simulink model "calibration_valves"  (R2026a)
settings: Solver=VariableStepAuto  StopTime=inf
InitFcn:
  | coefficients = [0,coefficients];
StopFcn:
  | az = out.az;
  | save(fullfile('calibration_data','az_calibration.mat'),'az');
settings Model: Creator=user  LastModifiedBy=jinyu

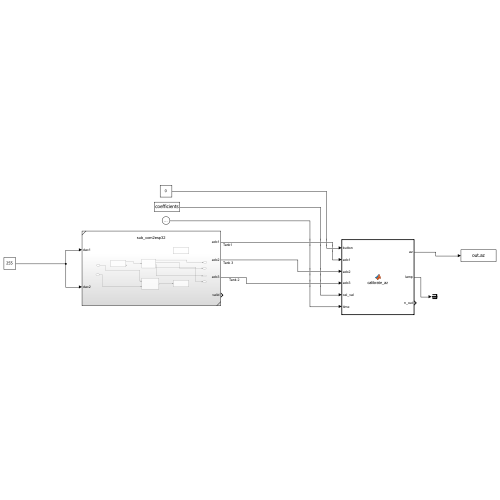
[thumbnail: Simulink's stored preview of the top-level diagram]
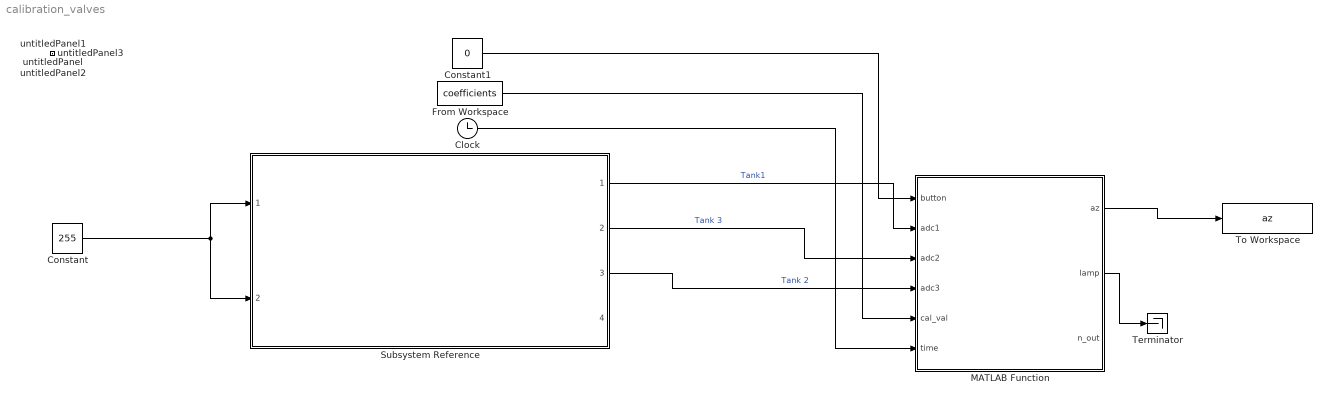
== system calibration_valves ==
  Clock : Clock
  Constant : Constant  Value=255
  Constant1 : Constant  Value=0
  From Workspace : FromWorkspace  VariableName=coefficients  SampleTime=-1
  MATLAB Function : MATLAB Function  TreatAsAtomicUnit=on
  Subsystem Reference : Subsystem  ReferencedSubsystem=sub_com2esp32
  Terminator : Terminator
  To Workspace : ToWorkspace  VariableName=az  SampleTime=-1
      settings: MaxDataPoints=1
  untitledPanel : Subsystem  Tag=HiddenForWebPanel  IsWebBlockPanel=on
  untitledPanel1 : Subsystem  Tag=HiddenForWebPanel  IsWebBlockPanel=on
  untitledPanel2 : Subsystem  Tag=HiddenForWebPanel  IsWebBlockPanel=on
  untitledPanel3 : Subsystem  Tag=HiddenForWebPanel  IsWebBlockPanel=on
  wires:
  Subsystem Reference/1 -> MATLAB Function/2(adc1)  "Tank1"
  MATLAB Function/1(az) -> To Workspace/1
  Constant/1 -> Subsystem Reference/2, Subsystem Reference/1
  From Workspace/1 -> MATLAB Function/5(cal_val)
  Clock/1 -> MATLAB Function/6(time)
  Constant1/1 -> MATLAB Function/1(button)
  Subsystem Reference/2 -> MATLAB Function/3(adc2)  "Tank 3"
  Subsystem Reference/3 -> MATLAB Function/4(adc3)  "Tank 2"
  MATLAB Function/2(lamp) -> Terminator/1

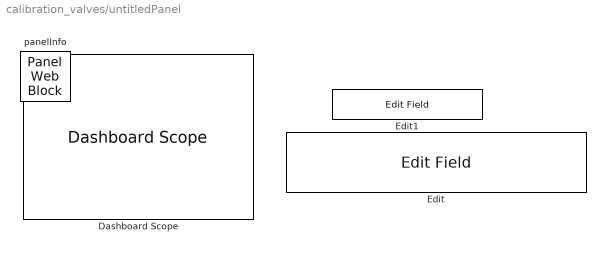
== system calibration_valves/untitledPanel ==
  Dashboard Scope : DashboardScope  Tag=HiddenForWebPanel  PanelInfo="{\"height\":195,\"left\":22,\"panelId\":\"panelId-0a8f6d05-5e0e-4052-8464-4cdde78ccbfe\",\"top\":22,\"type\":\"panelChild\",\"version\":\"2019b\",\"width\":271,\"zIndex\":1500002}"  FontColor=[0.0, 0.0, 0.0]
  Edit : EditField  Tag=HiddenForWebPanel  PanelInfo="{\"height\":25,\"left\":322,\"panelId\":\"panelId-0a8f6d05-5e0e-4052-8464-4cdde78ccbfe\",\"top\":100,\"type\":\"panelChild\",\"version\":\"2019b\",\"width\":181,\"zIndex\":1500006}"  LabelPosition=Hide  ShowInitialText=on  Alignment=Center
  Edit1 : EditField  Tag=HiddenForWebPanel  PanelInfo="{\"height\":30,\"left\":327,\"panelId\":\"panelId-0a8f6d05-5e0e-4052-8464-4cdde78ccbfe\",\"top\":53,\"type\":\"panelChild\",\"version\":\"2019b\",\"width\":150,\"zIndex\":1500004}"  LabelPosition=Hide  ShowInitialText=on  Alignment=Center
  panelInfo : PanelWebBlock  Tag=HiddenForWebPanel  PanelInfo="{\"compacted\":false,\"height\":362,\"isActiveTab\":false,\"left\":183,\"name\":\"Panel\",\"panelId\":\"panelId-0a8f6d05-5e0e-4052-8464-4cdde78ccbfe\",\"popoutData\":{\"height\":495,\"left\":546,\"maximized\":false,\"top\":827,\"width\":618},\"popoutMode\":\"windowHidden\",\"tabIndex\":0,\"tabbedSetId\":\"tabbedSet4972758365\",\"top\":737,\"type\":\"panel\",\"version\":\"2019b\",\"visible\":false,\"width\":602,\"zIndex\":1500002}"  PanelSnapshot=<binary blob, 20028 chars, not shown>

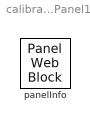
== system calibration_valves/untitledPanel1 ==
  panelInfo : PanelWebBlock  Tag=HiddenForWebPanel  PanelInfo="{\"compacted\":false,\"height\":362,\"isActiveTab\":true,\"left\":183,\"name\":\"Panel1\",\"panelId\":\"panelId-b2ee2f41-7720-49f1-b51a-3062c351f597\",\"popoutData\":{\"height\":495,\"left\":546,\"maximized\":false,\"top\":827,\"width\":618},\"popoutMode\":\"windowHidden\",\"tabIndex\":1,\"tabbedSetId\":\"tabbedSet4972758365\",\"top\":737,\"type\":\"panel\",\"version\":\"2019b\",\"visible\":true,\"width\":602,\"zIndex\":1500004}"

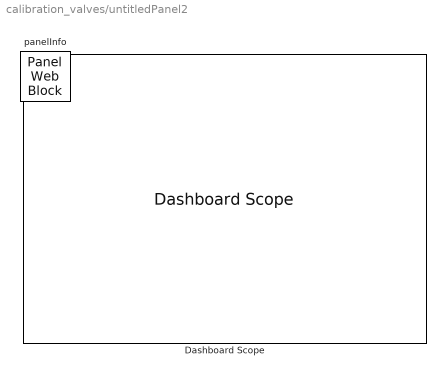
== system calibration_valves/untitledPanel2 ==
  Dashboard Scope : DashboardScope  Tag=HiddenForWebPanel  PanelInfo="{\"height\":289,\"left\":18,\"panelId\":\"panelId-8ba459e9-7eb9-43d1-9a8b-2b7bff5a2d5c\",\"top\":18,\"type\":\"panelChild\",\"version\":\"2019b\",\"width\":403,\"zIndex\":1500002}"  FontColor=[0.0, 0.0, 0.0]
  panelInfo : PanelWebBlock  Tag=HiddenForWebPanel  PanelInfo="{\"compacted\":false,\"height\":329,\"isActiveTab\":true,\"left\":1320,\"name\":\"Panel2\",\"panelId\":\"panelId-8ba459e9-7eb9-43d1-9a8b-2b7bff5a2d5c\",\"popoutData\":{\"height\":440,\"left\":1683,\"maximized\":false,\"top\":822,\"width\":459},\"popoutMode\":\"windowHidden\",\"tabIndex\":0,\"tabbedSetId\":\"tabbedSet1724704130\",\"top\":710,\"type\":\"panel\",\"version\":\"2019b\",\"visible\":true,\"width\":443,\"zIndex\":1500006}"  PanelSnapshot=<binary blob, 75208 chars, not shown>

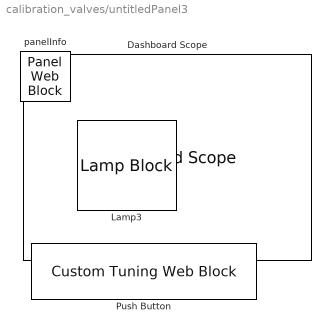
== system calibration_valves/untitledPanel3 ==
  Dashboard Scope : DashboardScope  Tag=HiddenForWebPanel  PanelInfo="{\"height\":461,\"left\":236,\"panelId\":\"panelId-037cc253-1a0e-430c-bfc3-d197bdfa8fb6\",\"top\":13,\"type\":\"panelChild\",\"version\":\"2019b\",\"width\":556,\"zIndex\":1500002}"  FontColor=[0.0, 0.0, 0.0]
  Lamp3 : LampBlock  Tag=HiddenForWebPanel  PanelInfo="{\"height\":68,\"left\":30,\"panelId\":\"panelId-037cc253-1a0e-430c-bfc3-d197bdfa8fb6\",\"top\":30,\"type\":\"panelChild\",\"version\":\"2019b\",\"width\":79,\"zIndex\":1500014}"  LabelPosition=Hide  DefaultColor=[192.0, 192.0, 192.0]
  Push Button : CustomTuningWebBlock  Tag=HiddenForWebPanel  PanelInfo="{\"height\":52,\"left\":27,\"panelId\":\"panelId-037cc253-1a0e-430c-bfc3-d197bdfa8fb6\",\"top\":105,\"type\":\"panelChild\",\"version\":\"2019b\",\"width\":209,\"zIndex\":1500008}"  LabelPosition=Hide  ShowInitialText=on  Configuration="{\"components\":[{\"name\":\"BackgroundImageComponent\",\"settings\":{\"image\":{\"size\":[0,0],\"src\":\"default\",\"srcOrientation\":\"horizontal\"},\"position\":[0,0,1,1],\"scaleMode\":\"0\"}},{\"name\":\"ButtonStateComponent\",\"settings\":{\"buttonType\":\"momentary\",\"clickFcn\":\"\",\"image\":{\"size\":[180,45],\"srcOrientation\":\"Right\"},\"latched\":false,\"offValue\":[],\"onValue\":1,\"position\":[0,0,1,1],\"pressDelay\":500,\"pressFcn\":\"\",\"repeatInterval\":0,\"states\":[{\"horizontalAlignment\":\"center\",\"image\":{\"position\":[0.05,0.015,0.98,0.9],\"size\":[0.98,0.9],\"src\":\"data:image\\/svg+xml;base64,PHN2ZyB4bWxucz0iaHR0cDovL3d3dy53My5vcmcvMjAwMC9zdmciIHhtbG5zOnhsaW5rPSJodHRwOi8vd3d3LnczLm9yZy8xOTk5L3hsaW5rIiB2aWV3Qm94PSIwIDAgMTc3LjI1IDQwLjg4Ij48ZGVmcz48c3R5bGU+LmNscy0xe2ZpbGw6dXJsKCNyYWRpYWwtZ3JhZGllbnQpO30uY2xzLTJ7ZmlsbDp1cmwoI2xpbmVhci1ncmFkaWVudCk7fS5jbHMtM3tmaWxsOnVybCgjbGluZWFyLWdyYWRpZW50LTIpO308L3N0eWxlPjxyYWRpYWxHcmFkaWVudCBpZD0icmFkaWFsLWdyYWRpZW50IiBjeD0iOTAuMDkiIGN5PSIyMi42NiIgcj0i ...(+2212 chars)\",\"srcOrientation\":\"Right\"},\"label\":{\"color\":[1,1,0.78,1],\"icon\":{\"size\":[1.2,1.2],\"src\":\"data:image\\/svg+xml;base64,PHN2ZyBpZD0iT2ZmIiB4bWxucz0iaHR0cDovL3d3dy53My5vcmcvMjAwMC9zdmciIHhtbG5zOnhsaW5rPSJodHRwOi8vd3d3LnczLm9yZy8xOTk5L3hsaW5rIiB2aWV3Qm94PSIwIDAgNTAgNTAiPjxkZWZzPjxzdHlsZT4uY2xzLTF7ZmlsbDojN2Y4MDgwO3N0cm9rZTojMjcyNjI2O3N0cm9rZS1taXRlcmxpbWl0OjEwO3N0cm9rZS13aWR0aDozcHg7fS5jbHMtMntmaWxsOnVybCgjbGluZWFyLWdyYWRpZW50KTt9PC9zdHlsZT48bGluZWFyR3JhZGllbnQgaWQ9ImxpbmVhci1ncmFkaWVudCIgeDE9IjI1IiB5MT0iOSIgeDI9IjI1IiB5Mj0iMzciIGdyYWRpZW50VW5pdHM9InVzZXJTcGFjZU9uVXNlIj48c3RvcCBvZmZzZXQ9IjAiIHN0b3AtY29sb3I9IiNmZmYiIHN0b3Atb3BhY2l0eT0iMC43NSIvPjxzdG9wIG9mZnNldD0iMSIgc3RvcC1jb2xvcj0iI2ZmZiIgc3RvcC1vcGFjaXR5PSIwIi8+PC9saW5lYXJHcmFkaWVudD48L2RlZnM+PGNpcmNsZSBjbGFzcz0iY2xzLTEiIGN4PSIyNSIgY3k9IjI1IiByPSIyMCIvPjxjaXJjbGUgY2xhc3M9ImNscy0yIiBjeD0iMjUiIGN5PSIyMyIgcj0iMTQiLz48L3N2Zz4=\",\"srcOrientation\":\"Right\"},\"iconOffset\":0,\"iconPlacement\":\"left\",\"opacity\":1,\"show\":true,\"text\":{\"content\":\"Button\",\"font\":\"Helvetica\"}},\"labelOffset\":[-0.025,0],\"verticalAlignment\":\"middle\"},{\"horizontalAlignment\":\"center\",\"image\":{\"position\":[0.05,0.015,0.98,0.9],\"size\":[0.98,0.9],\"src\":\"data:image\\/svg+xml;base64,PHN2ZyB4bWxucz0iaHR0cDovL3d3dy53My5vcmcvMjAwMC9zdmciIHhtbG5zOnhsaW5rPSJodHRwOi8vd3d3LnczLm9yZy8xOTk5L3hsaW5rIiB2aWV3Qm94PSIwIDAgMTc3LjI1IDQwLjg4Ij48ZGVmcz48c3R5bGU+LmNscy0xe2ZpbGw6dXJsKCNyYWRpYWwtZ3JhZGllbnQpO30uY2xzLTJ7ZmlsbDp1cmwoI2xpbmVhci1ncmFkaWVudCk7fS5jbHMtM3tmaWxsOnVybCgjbGluZWFyLWdyYWRpZW50LTIpO308L3N0eWxlPjxyYWRpYWxHcmFkaWVudCBpZD0icmFkaWFsLWdyYWRpZW50IiBjeD0iOTAuMDkiIGN5PSIyMi42NiIgcj0i ...(+2216 chars)\",\"srcOrientation\":\"Right\"},\"label\":{\"color\":[1,1,0.78,1],\"icon\":{\"size\":[1.2,1.2],\"src\":\"data:image\\/svg+xml;base64,PHN2ZyB4bWxucz0iaHR0cDovL3d3dy53My5vcmcvMjAwMC9zdmciIHhtbG5zOnhsaW5rPSJodHRwOi8vd3d3LnczLm9yZy8xOTk5L3hsaW5rIiB2aWV3Qm94PSIwIDAgNTAgNTAiPjxkZWZzPjxzdHlsZT4uY2xzLTF7ZmlsbDojNmFiZDQ1O3N0cm9rZTojMjcyNjI2O3N0cm9rZS1taXRlcmxpbWl0OjEwO3N0cm9rZS13aWR0aDozcHg7fS5jbHMtMntmaWxsOnVybCgjbGluZWFyLWdyYWRpZW50KTt9PC9zdHlsZT48bGluZWFyR3JhZGllbnQgaWQ9ImxpbmVhci1ncmFkaWVudCIgeDE9IjI1IiB5MT0iOSIgeDI9IjI1IiB5Mj0iMzciIGdyYWRpZW50VW5pdHM9InVzZXJTcGFjZU9uVXNlIj48c3RvcCBvZmZzZXQ9IjAiIHN0b3AtY29sb3I9IiNmZmYiIHN0b3Atb3BhY2l0eT0iMC43NSIvPjxzdG9wIG9mZnNldD0iMSIgc3RvcC1jb2xvcj0iI2ZmZiIgc3RvcC1vcGFjaXR5PSIwIi8+PC9saW5lYXJHcmFkaWVudD48L2RlZnM+PGcgaWQ9Ik9uIj48Y2lyY2xlIGNsYXNzPSJjbHMtMSIgY3g9IjI1IiBjeT0iMjUiIHI9IjIwIi8+PGNpcmNsZSBjbGFzcz0iY2xzLTIiIGN4PSIyNSIgY3k9IjIzIiByPSIxNCIvPjwvZz48L3N2Zz4=\",\"srcOrientation\":\"Right\"},\"iconOffset\":0,\"iconPlacement\":\"left\",\"opacity\":1,\"show\":true,\"text\":{\"content\":\"Button\",\"font\":\"Helvetica\"}},\"labelOffset\":[0,0],\"verticalAlignment\":\"middle\"},{\"horizontalAlignment\":\"center\",\"image\":{\"position\":[0.05,0.015,0.98,0.9],\"size\":[0.98,0.9],\"src\":\"data:image\\/svg+xml;base64,PHN2ZyB4bWxucz0iaHR0cDovL3d3dy53My5vcmcvMjAwMC9zdmciIHhtbG5zOnhsaW5rPSJodHRwOi8vd3d3LnczLm9yZy8xOTk5L3hsaW5rIiB2aWV3Qm94PSIwIDAgMTc3LjI1IDQwLjg4Ij48ZGVmcz48c3R5bGU+LmNscy0xe2ZpbGw6dXJsKCNyYWRpYWwtZ3JhZGllbnQpO30uY2xzLTJ7ZmlsbDp1cmwoI2xpbmVhci1ncmFkaWVudCk7fS5jbHMtM3tmaWxsOnVybCgjbGluZWFyLWdyYWRpZW50LTIpO308L3N0eWxlPjxyYWRpYWxHcmFkaWVudCBpZD0icmFkaWFsLWdyYWRpZW50IiBjeD0iOTAuMDkiIGN5PSIyMi42NiIgcj0i ...(+2212 chars)\",\"srcOrientation\":\"Right\"},\"label\":{\"color\":[1,1,0.78,1],\"icon\":{\"size\":[1.2,1.2],\"src\":\"data:image\\/svg+xml;base64,PHN2ZyB4bWxucz0iaHR0cDovL3d3dy53My5vcmcvMjAwMC9zdmciIHhtbG5zOnhsaW5rPSJodHRwOi8vd3d3LnczLm9yZy8xOTk5L3hsaW5rIiB2aWV3Qm94PSIwIDAgNTAgNTAiPjxkZWZzPjxzdHlsZT4uY2xzLTF7ZmlsbDojNmFiZDQ1O3N0cm9rZTojMjcyNjI2O3N0cm9rZS1taXRlcmxpbWl0OjEwO3N0cm9rZS13aWR0aDozcHg7fS5jbHMtMntmaWxsOnVybCgjbGluZWFyLWdyYWRpZW50KTt9PC9zdHlsZT48bGluZWFyR3JhZGllbnQgaWQ9ImxpbmVhci1ncmFkaWVudCIgeDE9IjI1IiB5MT0iOSIgeDI9IjI1IiB5Mj0iMzciIGdyYWRpZW50VW5pdHM9InVzZXJTcGFjZU9uVXNlIj48c3RvcCBvZmZzZXQ9IjAiIHN0b3AtY29sb3I9IiNmZmYiIHN0b3Atb3BhY2l0eT0iMC43NSIvPjxzdG9wIG9mZnNldD0iMSIgc3RvcC1jb2xvcj0iI2ZmZiIgc3RvcC1vcGFjaXR5PSIwIi8+PC9saW5lYXJHcmFkaWVudD48L2RlZnM+PGcgaWQ9Ik9uIj48Y2lyY2xlIGNsYXNzPSJjbHMtMSIgY3g9IjI1IiBjeT0iMjUiIHI9IjIwIi8+PGNpcmNsZSBjbGFzcz0iY2xzLTIiIGN4PSIyNSIgY3k9IjIzIiByPSIxNCIvPjwvZz48L3N2Zz4=\",\"srcOrientation\":\"Right\"},\"iconOffset\":0,\"iconPlacement\":\"left\",\"opacity\":1,\"show\":true,\"text\":{\"content\":\"Button\",\"font\":\"Helvetica\"}},\"labelOffset\":[-0.025,0],\"verticalAlignment\":\"middle\"},{\"horizontalAlignment\":\"center\",\"image\":{\"position\":[0.05,0.015,0.98,0.9],\"size\":[0.98,0.9],\"src\":\"data:image\\/svg+xml;base64,PHN2ZyB4bWxucz0iaHR0cDovL3d3dy53My5vcmcvMjAwMC9zdmciIHhtbG5zOnhsaW5rPSJodHRwOi8vd3d3LnczLm9yZy8xOTk5L3hsaW5rIiB2aWV3Qm94PSIwIDAgMTc3LjI1IDQwLjg4Ij48ZGVmcz48c3R5bGU+LmNscy0xe2ZpbGw6dXJsKCNyYWRpYWwtZ3JhZGllbnQpO30uY2xzLTJ7ZmlsbDp1cmwoI2xpbmVhci1ncmFkaWVudCk7fS5jbHMtM3tmaWxsOnVybCgjbGluZWFyLWdyYWRpZW50LTIpO308L3N0eWxlPjxyYWRpYWxHcmFkaWVudCBpZD0icmFkaWFsLWdyYWRpZW50IiBjeD0iOTAuMDkiIGN5PSIyMi42NiIgcj0i ...(+2216 chars)\",\"srcOrientation\":\"Right\"},\"label\":{\"color\":[1,1,0.78,1],\"icon\":{\"size\":[1.2,1.2],\"src\":\"data:image\\/svg+xml;base64,PHN2ZyBpZD0iT2ZmIiB4bWxucz0iaHR0cDovL3d3dy53My5vcmcvMjAwMC9zdmciIHhtbG5zOnhsaW5rPSJodHRwOi8vd3d3LnczLm9yZy8xOTk5L3hsaW5rIiB2aWV3Qm94PSIwIDAgNTAgNTAiPjxkZWZzPjxzdHlsZT4uY2xzLTF7ZmlsbDojN2Y4MDgwO3N0cm9rZTojMjcyNjI2O3N0cm9rZS1taXRlcmxpbWl0OjEwO3N0cm9rZS13aWR0aDozcHg7fS5jbHMtMntmaWxsOnVybCgjbGluZWFyLWdyYWRpZW50KTt9PC9zdHlsZT48bGluZWFyR3JhZGllbnQgaWQ9ImxpbmVhci1ncmFkaWVudCIgeDE9IjI1IiB5MT0iOSIgeDI9IjI1IiB5Mj0iMzciIGdyYWRpZW50VW5pdHM9InVzZXJTcGFjZU9uVXNlIj48c3RvcCBvZmZzZXQ9IjAiIHN0b3AtY29sb3I9IiNmZmYiIHN0b3Atb3BhY2l0eT0iMC43NSIvPjxzdG9wIG9mZnNldD0iMSIgc3RvcC1jb2xvcj0iI2ZmZiIgc3RvcC1vcGFjaXR5PSIwIi8+PC9saW5lYXJHcmFkaWVudD48L2RlZnM+PGNpcmNsZSBjbGFzcz0iY2xzLTEiIGN4PSIyNSIgY3k9IjI1IiByPSIyMCIvPjxjaXJjbGUgY2xhc3M9ImNscy0yIiBjeD0iMjUiIGN5PSIyMyIgcj0iMTQiLz48L3N2Zz4=\",\"srcOrientation\":\"Right\"},\"iconOffset\":0,\"iconPlacement\":\"left\",\"opacity\":1,\"show\":true,\"text\":{\"content\":\"Button\",\"font\":\"Helvetica\"}},\"labelOffset\":[0,0],\"verticalAlignment\":\"middle\"}]}},{\"name\":\"ForegroundImageComponent\",\"settings\":{\"image\":{\"size\":[0,0],\"src\":\"default\",\"srcOrientation\":\"horizontal\"},\"isForeground\":1,\"position\":[0,0,1,1],\"scaleMode\":\"0\"}}],\"derived\":{\"blockParameters\":{\"AutoActivate\":false,\"ButtonText\":\"Button\",\"ButtonType\":\"Momentary\",\"ClickFcn\":\"\",\"OnValue\":1,\"PressDelay\":500,\"PressFcn\":\"\",\"RepeatInterval\":0,\"fixedAspectRatio\":\"on\"}},\"settings\":{\"BindingType\":\"param\",\"aspectRatio\":3.7777777777777777,\"autoActivate\":false,\"backgroundColor\":[0,0,0,\"1\"],\"backgroundOffset\":0,\"backgroundOpacity\":1,\"fixedAspectRatio\":\"on\",\"foregroundColor\":[252,252,196],\"showBackgroundColor\":false,\"variant\":\"push\",\"version\":\"R2025a\"},\"type\":\"Button\"}"
  panelInfo : PanelWebBlock  Tag=HiddenForWebPanel  PanelInfo="{\"compacted\":true,\"height\":495,\"isActiveTab\":true,\"labels\":{},\"left\":630,\"name\":\"Panel3\",\"panelId\":\"panelId-037cc253-1a0e-430c-bfc3-d197bdfa8fb6\",\"tabIndex\":0,\"tabbedSetId\":\"tabbedSet3591606152\",\"top\":454,\"type\":\"panel\",\"version\":\"2019b\",\"visible\":true,\"width\":798,\"zIndex\":1500008}"  PanelSnapshot=<binary blob, 34728 chars, not shown>

== matlab function calibration_valves/MATLAB Function ==
  data: button input; adc1 input; adc2 input; adc3 input; cal_val input; az output; lamp output; time input; n_out output
function [az, lamp, n_out] = calibrate_az(button, adc1, adc2, adc3, cal_val, time)

persistent running t_start h1p h2p h3p tp m1 m2 m3 n az_out

az    = zeros(3,1);
lamp  = 0.0;
n_out = 0.0;

if isempty(running)
    running = 0.0;
    t_start = 0.0;
    h1p    = 0.0; h2p = 0.0; h3p = 0.0;
    tp     = 0.0;
    m1     = 0.0; m2  = 0.0; m3  = 0.0;
    n      = 0.0;
    az_out = zeros(3,1);
end

% Parameters all in cm
A  = 154.0;
Sn = 0.5;
g  = 981.0;

% T1=adc1, T2=adc3, T3=adc2
h1 = adc1(1) * cal_val(1);
h2 = adc3(1) * cal_val(1);
h3 = adc2(1) * cal_val(1);
t  = time(1);
b  = button(1);

% Only start if all tanks sufficiently filled
if b == 1 && running == 0 && h1 > 5 && h2 > 5 && h3 > 5
    running = 1.0;
    t_start = t;
    h1p = h1; h2p = h2; h3p = h3;
    tp  = t;
    m1  = 0.0; m2 = 0.0; m3 = 0.0;
    n   = 0.0;
end

if running == 1
    lamp = 1.0;
    dt   = t - tp;

    if dt > 0
        % Derivatives
        dh1 = (h1 - h1p) / dt;
        dh2 = (h2 - h2p) / dt;
        dh3 = (h3 - h3p) / dt;

        % Midpoint levels
        h1m = (h1 + h1p) / 2;
        h2m = (h2 + h2p) / 2;
        h3m = (h3 + h3p) / 2;

        % Potential flows (without az)
        Q13 = Sn * sqrt(2*g * max(h1m - h3m, 0));
        Q32 = Sn * sqrt(2*g * max(h3m - h2m, 0));
        Q20 = Sn * sqrt(2*g * max(h2m,       0));

        if Q13 > 0.001 && Q32 > 0.001 && Q20 > 0.001
            n   = n + 1;

            % Sequential solve
            az1 = (-dh1*A) / Q13;
            az3 = (az1*Q13 - dh3*A) / Q32;
            az2 = (az3*Q32 - dh2*A) / Q20;

            % Running mean
            m1 = (m1*(n-1) + az1) / n;
            m3 = (m3*(n-1) + az3) / n;
            m2 = (m2*(n-1) + az2) / n;
        end

        az_out(1) = m1;
        az_out(2) = m2;
        az_out(3) = m3;

        h1p = h1; h2p = h2; h3p = h3;
        tp  = t;
    end

    if (t - t_start) >= 60
        running = 2.0;
    end
end

if running == 2
    lamp = 2.0;
end

az    = az_out;
n_out = n;
